simulink model "sanxiangbanbokekongzhengliu"  (Simulink 7.3)
settings: Solver=ode15s  StartTime=0.0  StopTime=0.1  MaxStep=0.0000001  RelTol=1e-3
libraries: powerlib x10
settings Model: Creator=Administrator  LastModifiedBy=Administrator

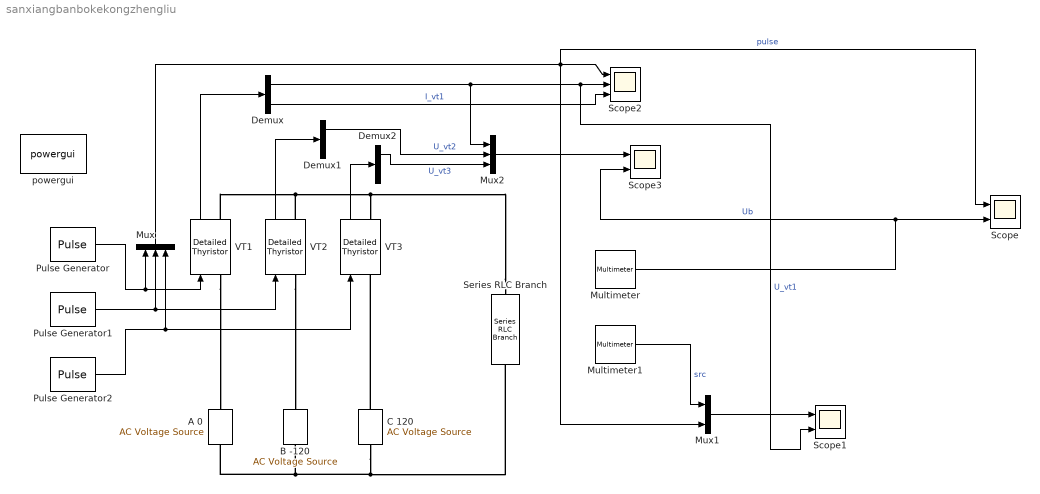
== system sanxiangbanbokekongzhengliu ==
  A 0 : powerlib/Electrical Sources/AC Voltage Source  DialogController=POWERSYS.PowerSysDialog  SystemSampleTime=-1  Amplitude=220  Phase=0  Frequency=50  SampleTime=0  Measurements=Voltage
  B -120 : powerlib/Electrical Sources/AC Voltage Source  DialogController=POWERSYS.PowerSysDialog  SystemSampleTime=-1  Amplitude=220  Phase=240  Frequency=50  SampleTime=0  Measurements=Voltage
  C 120 : powerlib/Electrical Sources/AC Voltage Source  DialogController=POWERSYS.PowerSysDialog  SystemSampleTime=-1  Amplitude=220  Phase=120  Frequency=50  SampleTime=0  Measurements=Voltage
  Demux : Demux  Outputs=2
  Demux1 : Demux  Outputs=2
  Demux2 : Demux  Outputs=2
  Multimeter : powerlib/Measurements/Multimeter  SystemSampleTime=-1  PhasorSimulation=off  OutputType=Complex  sel=1  L=5  Gain=1  yselected={'Ub: Series RLC Branch'};  PSBOutputType=1  PSBequivalent=0  AxesSetting=[0,0.1,-100,100]  Display=0  SavedBlockNames=-11
  Multimeter1 : powerlib/Measurements/Multimeter  SystemSampleTime=-1  PhasorSimulation=off  OutputType=Complex  sel=[3 4 2]  L=5  Gain=[1 1 1]  yselected={'Usrc: A 0','Usrc: B -120','Usrc: C 120'};  PSBOutputType=1  PSBequivalent=0  AxesSetting=[0,0.1,-100,100]  Display=0  SavedBlockNames=-11
  Mux : Mux  Inputs=3
  Mux1 : Mux  Inputs=2
  Mux2 : Mux  Inputs=3
  Pulse Generator : DiscretePulseGenerator  PulseType=Time based  Amplitude=10  Period=0.02  PulseWidth=5  PhaseDelay=0.003277  SampleTime=1
  Pulse Generator1 : DiscretePulseGenerator  PulseType=Time based  Amplitude=10  Period=0.02  PulseWidth=5  PhaseDelay=0.00994  SampleTime=1
  Pulse Generator2 : DiscretePulseGenerator  PulseType=Time based  Amplitude=10  Period=0.02  PulseWidth=5  PhaseDelay=0.016611  SampleTime=1
  Scope : Scope  NumInputPorts=2
      settings: YMin=0~-10  YMax=10~220
  Scope1 : Scope  NumInputPorts=2
      settings: YMin=-225~-1  YMax=225~22
  Scope2 : Scope  NumInputPorts=3
      settings: YMin=-20~-5~-5  YMax=20~5~5  SaveName=ScopeData2
  Scope3 : Scope  NumInputPorts=2
      settings: YMin=-5~-5  YMax=5~5  SaveName=ScopeData3
  Series RLC Branch : powerlib/Elements/Series RLC Branch  DialogController=POWERSYS.PowerSysDialog  PhysicalDomain=powersysdomain  SubClassName=unknown  LeftPortType=p1  RightPortType=p1  LConnTagsString=__new0  RConnTagsString=__new0  BranchType=R  Resistance=10  Inductance=1e-3  SetiL0=off  InitialCurrent=0  Capacitance=1e-6  Setx0=off  InitialVoltage=0  Measurements=Branch voltage and current
  VT1 : powerlib/Power Electronics/Detailed Thyristor  DialogController=POWERSYS.PowerSysDialog  SystemSampleTime=-1  Ron=0.001  Lon=1e-3  Vf=0.8  IL=0.1  Tq=100e-6  IC=0  Rs=500  Cs=250e-9  Measurements=on
  VT2 : powerlib/Power Electronics/Detailed Thyristor  DialogController=POWERSYS.PowerSysDialog  SystemSampleTime=-1  Ron=0.001  Lon=1e-3  Vf=0.8  IL=0.1  Tq=100e-6  IC=0  Rs=500  Cs=250e-9  Measurements=on
  VT3 : powerlib/Power Electronics/Detailed Thyristor  DialogController=POWERSYS.PowerSysDialog  SystemSampleTime=-1  Ron=0.001  Lon=1e-3  Vf=0.8  IL=0.1  Tq=100e-6  IC=0  Rs=500  Cs=250e-9  Measurements=on
  powergui : powerlib/powergui  Priority=1  SystemSampleTime=-1  SimulationMode=Continuous  SampleTime=50e-6  frequency=60  SPID=off  DisableSnubberDevices=off  DisableRonSwitches=off  DisableVfSwitches=off  SwTol=0  Interpol=off  frequencyindice=50  echomessages=off  HookPort=off  DisplayEquations=off  FunctionMessages=off  EnableUseOfTLC=off  x0status=blocks  RestoreLinks=warning  Frange=[0:2:500]  Ylog=off  Xlog=on  ShowGrid=off  save=off  variable=ZData  ZoomFFT=on  StartTime=0.0  cycles=1  DisplayStyle=1  fundamental=60  FreqAxis=off  MaxFrequency=1000  frequencyindicesteady=1  RmsSteady=1  display=off  Ts=0  methode=off
  wires:
  Pulse Generator/1 -> Mux/1, VT1/1
  Pulse Generator1/1 -> VT2/1, Mux/2
  Pulse Generator2/1 -> VT3/1, Mux/3
  VT1/1 -> Demux/1
  Demux/1 -> Scope2/2, Scope1/2, Mux2/1  "U_vt1"
  Demux/2 -> Scope2/3  "I_vt1"
  Mux/1 -> Scope2/1, Scope/1, Mux1/2  "pulse"
  Multimeter1/1 -> Mux1/1  "src"
  Mux1/1 -> Scope1/1
  VT2/1 -> Demux1/1
  VT3/1 -> Demux2/1
  Demux1/1 -> Mux2/2  "U_vt2"
  Demux2/1 -> Mux2/3  "U_vt3"
  Mux2/1 -> Scope3/1
  Multimeter/1 -> Scope/2, Scope3/2  "Ub"
  connections:
  Series RLC Branch/RConn1 -- C 120/LConn1 -- B -120/LConn1 -- A 0/LConn1
  Series RLC Branch/LConn1 -- VT1/RConn1 -- VT2/RConn1 -- VT3/RConn1
  VT1/LConn1 -- A 0/RConn1
  VT2/LConn1 -- B -120/RConn1
  C 120/RConn1 -- VT3/LConn1
